simulink model "FlightControlArchitecture"  (R2022a)
settings: Solver=VariableStepAuto  StartTime=0.0  StopTime=10.0  RelTol=1e-3
settings Model: Creator=pownc  LastModifiedBy=pownc

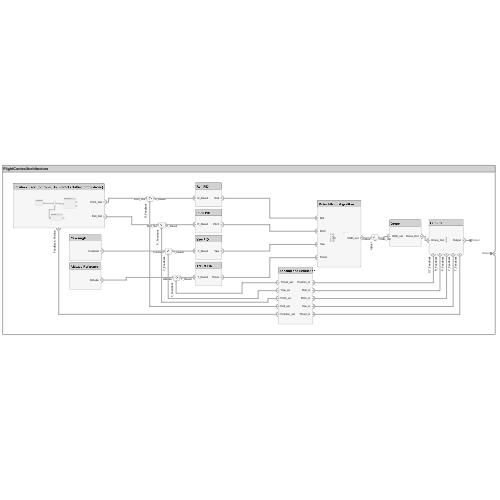
[thumbnail: Simulink's stored preview of the top-level diagram]
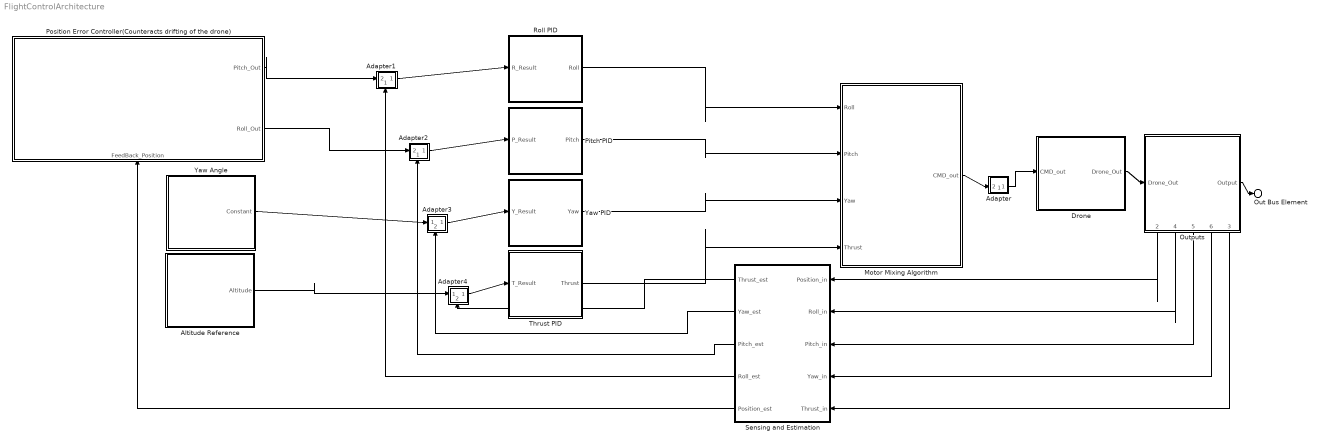
== system FlightControlArchitecture ==
  Adapter : Subsystem
      settings: PortSchema="{\"entries\":[{\"content\":{\"margin\":10,\"minimumSpacing\":15,\"sides\":[{\"content\":{\"connectorIds\":[\"In2\"]},\"type\":\"ConnectorPlacement.EquallySpacedRectSide\",\"uuid\":\"d6b19c1a-8540-4fb3-b3a7-b181a93e2dcd\"},{\"content\":{\"connectorIds\":[\"Out1\"],\"side\":\"RIGHT\"},\"type\":\"ConnectorPlacement.EquallySpacedRectSide\",\"uuid\":\"919fe610-1017-4d7e-ba89-b997ed30f941\"},{\"content\":{\"connectorIds\":[],\"side\":\"TOP\"},\"type\":\"ConnectorPlacement.EquallySpacedRectSide\",\"uuid\":\"6473f4db-e183-4279-8b70-07d1c7c027c3\"},{\"content\":{\"connectorIds\":[\"In1\"],\"side\":\"BOTTOM\"},\"type\":\"ConnectorPlacement.EquallySpacedRectSide\",\"uuid\":\"001743d6-53a9-4507-8ba9-ff0a8338509d\"}]},\"type\":\"ConnectorPlacement.EquallySpacedConnector\",\"uuid\":\"f0cd8fda-dd3e-48df-a1f9-a7820f464db5\"}],\"packageUris\":[\"http://schema.mathworks.com/mf0/Connector/R2020b\"],\"version\":\"1.0\"}"
  Adapter1 : Subsystem
      settings: PortSchema="{\"entries\":[{\"content\":{\"margin\":10,\"minimumSpacing\":15,\"sides\":[{\"content\":{\"connectorIds\":[\"In2\"]},\"type\":\"ConnectorPlacement.EquallySpacedRectSide\",\"uuid\":\"d6b19c1a-8540-4fb3-b3a7-b181a93e2dcd\"},{\"content\":{\"connectorIds\":[\"Out1\"],\"side\":\"RIGHT\"},\"type\":\"ConnectorPlacement.EquallySpacedRectSide\",\"uuid\":\"919fe610-1017-4d7e-ba89-b997ed30f941\"},{\"content\":{\"connectorIds\":[],\"side\":\"TOP\"},\"type\":\"ConnectorPlacement.EquallySpacedRectSide\",\"uuid\":\"6473f4db-e183-4279-8b70-07d1c7c027c3\"},{\"content\":{\"connectorIds\":[\"In1\"],\"side\":\"BOTTOM\"},\"type\":\"ConnectorPlacement.EquallySpacedRectSide\",\"uuid\":\"7437e3f3-5fc3-44ba-b792-8c2483ff9ea8\"}]},\"type\":\"ConnectorPlacement.EquallySpacedConnector\",\"uuid\":\"f0cd8fda-dd3e-48df-a1f9-a7820f464db5\"}],\"packageUris\":[\"http://schema.mathworks.com/mf0/Connector/R2020b\"],\"version\":\"1.0\"}"
  Adapter2 : Subsystem
      settings: PortSchema="{\"entries\":[{\"content\":{\"margin\":10,\"minimumSpacing\":15,\"sides\":[{\"content\":{\"connectorIds\":[\"In2\"]},\"type\":\"ConnectorPlacement.EquallySpacedRectSide\",\"uuid\":\"d6b19c1a-8540-4fb3-b3a7-b181a93e2dcd\"},{\"content\":{\"connectorIds\":[\"Out1\"],\"side\":\"RIGHT\"},\"type\":\"ConnectorPlacement.EquallySpacedRectSide\",\"uuid\":\"919fe610-1017-4d7e-ba89-b997ed30f941\"},{\"content\":{\"connectorIds\":[],\"side\":\"TOP\"},\"type\":\"ConnectorPlacement.EquallySpacedRectSide\",\"uuid\":\"6473f4db-e183-4279-8b70-07d1c7c027c3\"},{\"content\":{\"connectorIds\":[\"In1\"],\"side\":\"BOTTOM\"},\"type\":\"ConnectorPlacement.EquallySpacedRectSide\",\"uuid\":\"a3707513-231b-4166-bb59-f1312184589a\"}]},\"type\":\"ConnectorPlacement.EquallySpacedConnector\",\"uuid\":\"f0cd8fda-dd3e-48df-a1f9-a7820f464db5\"}],\"packageUris\":[\"http://schema.mathworks.com/mf0/Connector/R2020b\"],\"version\":\"1.0\"}"
  Adapter3 : Subsystem
      settings: PortSchema="{\"entries\":[{\"content\":{\"margin\":10,\"minimumSpacing\":15,\"sides\":[{\"content\":{\"connectorIds\":[\"In1\"]},\"type\":\"ConnectorPlacement.EquallySpacedRectSide\",\"uuid\":\"d6b19c1a-8540-4fb3-b3a7-b181a93e2dcd\"},{\"content\":{\"connectorIds\":[\"Out1\"],\"side\":\"RIGHT\"},\"type\":\"ConnectorPlacement.EquallySpacedRectSide\",\"uuid\":\"919fe610-1017-4d7e-ba89-b997ed30f941\"},{\"content\":{\"connectorIds\":[],\"side\":\"TOP\"},\"type\":\"ConnectorPlacement.EquallySpacedRectSide\",\"uuid\":\"6473f4db-e183-4279-8b70-07d1c7c027c3\"},{\"content\":{\"connectorIds\":[\"In2\"],\"side\":\"BOTTOM\"},\"type\":\"ConnectorPlacement.EquallySpacedRectSide\",\"uuid\":\"50c041b2-6c26-49b7-bedc-5dbf061703b8\"}]},\"type\":\"ConnectorPlacement.EquallySpacedConnector\",\"uuid\":\"f0cd8fda-dd3e-48df-a1f9-a7820f464db5\"}],\"packageUris\":[\"http://schema.mathworks.com/mf0/Connector/R2020b\"],\"version\":\"1.0\"}"
  Adapter4 : Subsystem
      settings: PortSchema="{\"entries\":[{\"content\":{\"margin\":10,\"minimumSpacing\":15,\"sides\":[{\"content\":{\"connectorIds\":[\"In1\"]},\"type\":\"ConnectorPlacement.EquallySpacedRectSide\",\"uuid\":\"d6b19c1a-8540-4fb3-b3a7-b181a93e2dcd\"},{\"content\":{\"connectorIds\":[\"Out1\"],\"side\":\"RIGHT\"},\"type\":\"ConnectorPlacement.EquallySpacedRectSide\",\"uuid\":\"919fe610-1017-4d7e-ba89-b997ed30f941\"},{\"content\":{\"connectorIds\":[],\"side\":\"TOP\"},\"type\":\"ConnectorPlacement.EquallySpacedRectSide\",\"uuid\":\"6473f4db-e183-4279-8b70-07d1c7c027c3\"},{\"content\":{\"connectorIds\":[\"In2\"],\"side\":\"BOTTOM\"},\"type\":\"ConnectorPlacement.EquallySpacedRectSide\",\"uuid\":\"d02c2b55-2766-4554-926c-619c29dbf015\"}]},\"type\":\"ConnectorPlacement.EquallySpacedConnector\",\"uuid\":\"f0cd8fda-dd3e-48df-a1f9-a7820f464db5\"}],\"packageUris\":[\"http://schema.mathworks.com/mf0/Connector/R2020b\"],\"version\":\"1.0\"}"
  Altitude Reference : Subsystem
      settings: PortSchema="{\"entries\":[{\"content\":{\"headerSize\":26,\"margin\":15,\"minimumSpacing\":25,\"sides\":[{\"content\":{\"connectorIds\":[]},\"type\":\"ConnectorPlacement.EquallySpacedRectSide\",\"uuid\":\"d6b19c1a-8540-4fb3-b3a7-b181a93e2dcd\"},{\"content\":{\"connectorIds\":[\"Out1\"],\"side\":\"RIGHT\"},\"type\":\"ConnectorPlacement.EquallySpacedRectSide\",\"uuid\":\"919fe610-1017-4d7e-ba89-b997ed30f941\"},{\"content\":{\"connectorIds\":[],\"side\":\"TOP\"},\"type\":\"ConnectorPlacement.EquallySpacedRectSide\",\"uuid\":\"6473f4db-e183-4279-8b70-07d1c7c027c3\"}]},\"type\":\"ConnectorPlacement.EquallySpacedConnector\",\"uuid\":\"f0cd8fda-dd3e-48df-a1f9-a7820f464db5\"}],\"packageUris\":[\"http://schema.mathworks.com/mf0/Connector/R2020b\"],\"version\":\"1.0\"}"
  Drone : Subsystem
      settings: PortSchema="{\"entries\":[{\"content\":{\"headerSize\":26,\"margin\":15,\"minimumSpacing\":25,\"sides\":[{\"content\":{\"connectorIds\":[\"In1\"]},\"type\":\"ConnectorPlacement.EquallySpacedRectSide\",\"uuid\":\"d6b19c1a-8540-4fb3-b3a7-b181a93e2dcd\"},{\"content\":{\"connectorIds\":[\"Out1\"],\"side\":\"RIGHT\"},\"type\":\"ConnectorPlacement.EquallySpacedRectSide\",\"uuid\":\"919fe610-1017-4d7e-ba89-b997ed30f941\"},{\"content\":{\"connectorIds\":[],\"side\":\"TOP\"},\"type\":\"ConnectorPlacement.EquallySpacedRectSide\",\"uuid\":\"6473f4db-e183-4279-8b70-07d1c7c027c3\"}]},\"type\":\"ConnectorPlacement.EquallySpacedConnector\",\"uuid\":\"f0cd8fda-dd3e-48df-a1f9-a7820f464db5\"}],\"packageUris\":[\"http://schema.mathworks.com/mf0/Connector/R2020b\"],\"version\":\"1.0\"}"
  Motor Mixing Algorithm : Subsystem
      settings: PortSchema="{\"entries\":[{\"content\":{\"headerSize\":26,\"margin\":15,\"minimumSpacing\":25,\"sides\":[{\"content\":{\"connectorIds\":[\"In1\",\"In2\",\"In3\",\"In4\"]},\"type\":\"ConnectorPlacement.EquallySpacedRectSide\",\"uuid\":\"7a3b38b8-6f09-4e2e-ab1c-f7a95debc383\"},{\"content\":{\"connectorIds\":[\"Out1\"],\"side\":\"RIGHT\"},\"type\":\"ConnectorPlacement.EquallySpacedRectSide\",\"uuid\":\"c60604c7-2225-45b1-bf81-c4b0e619cd15\"},{\"content\":{\"connectorIds\":[],\"side\":\"TOP\"},\"type\":\"ConnectorPlacement.EquallySpacedRectSide\",\"uuid\":\"851cd2f2-1711-4180-941f-21dd02fa4550\"}]},\"type\":\"ConnectorPlacement.EquallySpacedConnector\",\"uuid\":\"5057f251-a455-43c7-b15c-b3d1f8a9e1a3\"}],\"packageUris\":[\"http://schema.mathworks.com/mf0/Connector/R2020b\"],\"version\":\"1.0\"}"
  Outputs : Subsystem
      settings: PortSchema="{\"entries\":[{\"content\":{\"headerSize\":26,\"margin\":15,\"minimumSpacing\":25,\"sides\":[{\"content\":{\"connectorIds\":[\"In1\"]},\"type\":\"ConnectorPlacement.EquallySpacedRectSide\",\"uuid\":\"d6b19c1a-8540-4fb3-b3a7-b181a93e2dcd\"},{\"content\":{\"connectorIds\":[\"Out1\"],\"side\":\"RIGHT\"},\"type\":\"ConnectorPlacement.EquallySpacedRectSide\",\"uuid\":\"919fe610-1017-4d7e-ba89-b997ed30f941\"},{\"content\":{\"connectorIds\":[],\"side\":\"TOP\"},\"type\":\"ConnectorPlacement.EquallySpacedRectSide\",\"uuid\":\"6473f4db-e183-4279-8b70-07d1c7c027c3\"},{\"content\":{\"connectorIds\":[\"Out2\",\"Out4\",\"Out5\",\"Out6\",\"Out3\"],\"side\":\"BOTTOM\"},\"type\":\"ConnectorPlacement.EquallySpacedRectSide\",\"uuid\":\"c79be452-f41b-4e6d-ad81-53eba8a6a323\"}]},\"type\":\"ConnectorPlacement.EquallySpacedConnector\",\"uuid\":\"f0cd8fda-dd3e-48df-a1f9-a7820f464db5\"}],\"packageUris\":[\"http://schema.mathworks.com/mf0/Connector/R2020b\"],\"version\":\"1.0\"}"
  Pitch PID : Subsystem
      settings: PortSchema="{\"entries\":[{\"content\":{\"headerSize\":26,\"margin\":15,\"minimumSpacing\":25,\"sides\":[{\"content\":{\"connectorIds\":[\"In1\"]},\"type\":\"ConnectorPlacement.EquallySpacedRectSide\",\"uuid\":\"d6b19c1a-8540-4fb3-b3a7-b181a93e2dcd\"},{\"content\":{\"connectorIds\":[\"Out1\"],\"side\":\"RIGHT\"},\"type\":\"ConnectorPlacement.EquallySpacedRectSide\",\"uuid\":\"919fe610-1017-4d7e-ba89-b997ed30f941\"},{\"content\":{\"connectorIds\":[],\"side\":\"TOP\"},\"type\":\"ConnectorPlacement.EquallySpacedRectSide\",\"uuid\":\"6473f4db-e183-4279-8b70-07d1c7c027c3\"}]},\"type\":\"ConnectorPlacement.EquallySpacedConnector\",\"uuid\":\"f0cd8fda-dd3e-48df-a1f9-a7820f464db5\"}],\"packageUris\":[\"http://schema.mathworks.com/mf0/Connector/R2020b\"],\"version\":\"1.0\"}"
  Position Error Controller(Counteracts drifting of the drone) : Subsystem
      settings: PortSchema="{\"entries\":[{\"content\":{\"headerSize\":26,\"margin\":15,\"minimumSpacing\":25,\"sides\":[{\"content\":{\"connectorIds\":[]},\"type\":\"ConnectorPlacement.EquallySpacedRectSide\",\"uuid\":\"d6b19c1a-8540-4fb3-b3a7-b181a93e2dcd\"},{\"content\":{\"connectorIds\":[\"Out1\",\"Out2\"],\"side\":\"RIGHT\"},\"type\":\"ConnectorPlacement.EquallySpacedRectSide\",\"uuid\":\"919fe610-1017-4d7e-ba89-b997ed30f941\"},{\"content\":{\"connectorIds\":[],\"side\":\"TOP\"},\"type\":\"ConnectorPlacement.EquallySpacedRectSide\",\"uuid\":\"6473f4db-e183-4279-8b70-07d1c7c027c3\"},{\"content\":{\"connectorIds\":[\"In1\"],\"side\":\"BOTTOM\"},\"type\":\"ConnectorPlacement.EquallySpacedRectSide\",\"uuid\":\"7201be1c-4784-47e8-b556-a6345fcdd719\"}]},\"type\":\"ConnectorPlacement.EquallySpacedConnector\",\"uuid\":\"f0cd8fda-dd3e-48df-a1f9-a7820f464db5\"}],\"packageUris\":[\"http://schema.mathworks.com/mf0/Connector/R2020b\"],\"version\":\"1.0\"}"
  Roll PID : Subsystem
      settings: PortSchema="{\"entries\":[{\"content\":{\"headerSize\":26,\"margin\":15,\"minimumSpacing\":25,\"sides\":[{\"content\":{\"connectorIds\":[\"In1\"]},\"type\":\"ConnectorPlacement.EquallySpacedRectSide\",\"uuid\":\"d6b19c1a-8540-4fb3-b3a7-b181a93e2dcd\"},{\"content\":{\"connectorIds\":[\"Out1\"],\"side\":\"RIGHT\"},\"type\":\"ConnectorPlacement.EquallySpacedRectSide\",\"uuid\":\"919fe610-1017-4d7e-ba89-b997ed30f941\"},{\"content\":{\"connectorIds\":[],\"side\":\"TOP\"},\"type\":\"ConnectorPlacement.EquallySpacedRectSide\",\"uuid\":\"6473f4db-e183-4279-8b70-07d1c7c027c3\"}]},\"type\":\"ConnectorPlacement.EquallySpacedConnector\",\"uuid\":\"f0cd8fda-dd3e-48df-a1f9-a7820f464db5\"}],\"packageUris\":[\"http://schema.mathworks.com/mf0/Connector/R2020b\"],\"version\":\"1.0\"}"
  Sensing and Estimation : Subsystem
      settings: PortSchema="{\"entries\":[{\"content\":{\"headerSize\":26,\"margin\":15,\"minimumSpacing\":25,\"sides\":[{\"content\":{\"connectorIds\":[\"Out1\",\"Out2\",\"Out3\",\"Out4\",\"Out5\"]},\"type\":\"ConnectorPlacement.EquallySpacedRectSide\",\"uuid\":\"d6b19c1a-8540-4fb3-b3a7-b181a93e2dcd\"},{\"content\":{\"connectorIds\":[\"In5\",\"In4\",\"In3\",\"In2\",\"In1\"],\"side\":\"RIGHT\"},\"type\":\"ConnectorPlacement.EquallySpacedRectSide\",\"uuid\":\"919fe610-1017-4d7e-ba89-b997ed30f941\"},{\"content\":{\"connectorIds\":[],\"side\":\"TOP\"},\"type\":\"ConnectorPlacement.EquallySpacedRectSide\",\"uuid\":\"6473f4db-e183-4279-8b70-07d1c7c027c3\"}]},\"type\":\"ConnectorPlacement.EquallySpacedConnector\",\"uuid\":\"f0cd8fda-dd3e-48df-a1f9-a7820f464db5\"}],\"packageUris\":[\"http://schema.mathworks.com/mf0/Connector/R2020b\"],\"version\":\"1.0\"}"
  Thrust PID : Subsystem
      settings: PortSchema="{\"entries\":[{\"content\":{\"headerSize\":26,\"margin\":15,\"minimumSpacing\":25,\"sides\":[{\"content\":{\"connectorIds\":[\"In1\"]},\"type\":\"ConnectorPlacement.EquallySpacedRectSide\",\"uuid\":\"d6b19c1a-8540-4fb3-b3a7-b181a93e2dcd\"},{\"content\":{\"connectorIds\":[\"Out1\"],\"side\":\"RIGHT\"},\"type\":\"ConnectorPlacement.EquallySpacedRectSide\",\"uuid\":\"919fe610-1017-4d7e-ba89-b997ed30f941\"},{\"content\":{\"connectorIds\":[],\"side\":\"TOP\"},\"type\":\"ConnectorPlacement.EquallySpacedRectSide\",\"uuid\":\"6473f4db-e183-4279-8b70-07d1c7c027c3\"}]},\"type\":\"ConnectorPlacement.EquallySpacedConnector\",\"uuid\":\"f0cd8fda-dd3e-48df-a1f9-a7820f464db5\"}],\"packageUris\":[\"http://schema.mathworks.com/mf0/Connector/R2020b\"],\"version\":\"1.0\"}"
  Yaw Angle : Subsystem
      settings: PortSchema="{\"entries\":[{\"content\":{\"headerSize\":26,\"margin\":15,\"minimumSpacing\":25,\"sides\":[{\"content\":{\"connectorIds\":[]},\"type\":\"ConnectorPlacement.EquallySpacedRectSide\",\"uuid\":\"d6b19c1a-8540-4fb3-b3a7-b181a93e2dcd\"},{\"content\":{\"connectorIds\":[\"Out1\"],\"side\":\"RIGHT\"},\"type\":\"ConnectorPlacement.EquallySpacedRectSide\",\"uuid\":\"919fe610-1017-4d7e-ba89-b997ed30f941\"},{\"content\":{\"connectorIds\":[],\"side\":\"TOP\"},\"type\":\"ConnectorPlacement.EquallySpacedRectSide\",\"uuid\":\"6473f4db-e183-4279-8b70-07d1c7c027c3\"}]},\"type\":\"ConnectorPlacement.EquallySpacedConnector\",\"uuid\":\"f0cd8fda-dd3e-48df-a1f9-a7820f464db5\"}],\"packageUris\":[\"http://schema.mathworks.com/mf0/Connector/R2020b\"],\"version\":\"1.0\"}"
  Yaw PID : Subsystem
      settings: PortSchema="{\"entries\":[{\"content\":{\"headerSize\":26,\"margin\":15,\"minimumSpacing\":25,\"sides\":[{\"content\":{\"connectorIds\":[\"In1\"]},\"type\":\"ConnectorPlacement.EquallySpacedRectSide\",\"uuid\":\"d6b19c1a-8540-4fb3-b3a7-b181a93e2dcd\"},{\"content\":{\"connectorIds\":[\"Out1\"],\"side\":\"RIGHT\"},\"type\":\"ConnectorPlacement.EquallySpacedRectSide\",\"uuid\":\"919fe610-1017-4d7e-ba89-b997ed30f941\"},{\"content\":{\"connectorIds\":[],\"side\":\"TOP\"},\"type\":\"ConnectorPlacement.EquallySpacedRectSide\",\"uuid\":\"6473f4db-e183-4279-8b70-07d1c7c027c3\"}]},\"type\":\"ConnectorPlacement.EquallySpacedConnector\",\"uuid\":\"f0cd8fda-dd3e-48df-a1f9-a7820f464db5\"}],\"packageUris\":[\"http://schema.mathworks.com/mf0/Connector/R2020b\"],\"version\":\"1.0\"}"
  Out Bus Element : Outport  PortName=Output
  wires:
  Roll PID/1(Roll) -> Motor Mixing Algorithm/1(Roll)
  Pitch PID/1(Pitch) -> Motor Mixing Algorithm/2(Pitch)
  Yaw PID/1(Yaw) -> Motor Mixing Algorithm/3(Yaw)
  Thrust PID/1(Thrust) -> Motor Mixing Algorithm/4(Thrust)
  Adapter/1(CMD_out) -> Drone/1(CMD_out)
  Motor Mixing Algorithm/1(CMD_out) -> Adapter/2(InBus)
  Position Error Controller(Counteracts drifting of the drone)/1(Pitch_Out) -> Adapter1/2(Pitch_Out)
  Drone/1(Drone_Out) -> Outputs/1(Drone_Out)
  Adapter4/1(T_Result) -> Thrust PID/1(T_Result)
  Position Error Controller(Counteracts drifting of the drone)/2(Roll_Out) -> Adapter2/2(Roll_Out)
  Adapter1/1(R_Result) -> Roll PID/1(R_Result)
  Adapter2/1(P_Result) -> Pitch PID/1(P_Result)
  Adapter3/1(Y_Result) -> Yaw PID/1(Y_Result)
  Outputs/1(Output) -> Out Bus Element/1
  Outputs/2(XY_Feedback) -> Sensing and Estimation/5(Position_in)
  Outputs/4(R_Feedback) -> Sensing and Estimation/4(Roll_in)
  Outputs/5(P_Feedback) -> Sensing and Estimation/3(Pitch_in)
  Outputs/6(Y_Feedback) -> Sensing and Estimation/2(Yaw_in)
  Outputs/3(T_Feedback) -> Sensing and Estimation/1(Thrust_in)
  Sensing and Estimation/1(Thrust_est) -> Adapter4/2(T_Feedback)
  Sensing and Estimation/2(Yaw_est) -> Adapter3/2(Y_Feedback)
  Sensing and Estimation/3(Pitch_est) -> Adapter2/1(P_Feedback)
  Sensing and Estimation/4(Roll_est) -> Adapter1/1(R_Feedback)
  Sensing and Estimation/5(Position_est) -> Position Error Controller(Counteracts drifting of the drone)/1(FeedBack_Position)
  Yaw Angle/1(Constant) -> Adapter3/1(Constant)
  Altitude Reference/1(Altitude) -> Adapter4/1(Altitude)

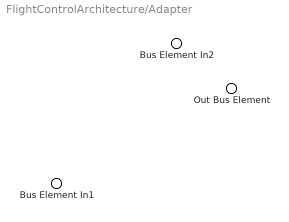
== system FlightControlArchitecture/Adapter ==
  Bus Element In2 : Inport  PortName=InBus1
  Bus Element In1 : Inport  Port=2  PortName=InBus
  Out Bus Element : Outport  PortName=CMD_out

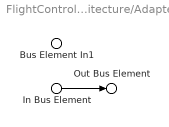
== system FlightControlArchitecture/Adapter1 ==
  Bus Element In1 : Inport  PortName=R_Feedback
  In Bus Element : Inport  Port=2  PortName=Pitch_Out
  Out Bus Element : Outport  PortName=R_Result
  wires:
  In Bus Element/1 -> Out Bus Element/1

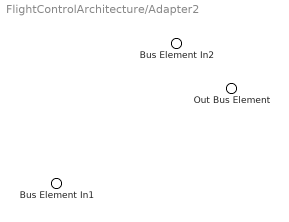
== system FlightControlArchitecture/Adapter2 ==
  Bus Element In2 : Inport  PortName=P_Feedback
  Bus Element In1 : Inport  Port=2  PortName=Roll_Out
  Out Bus Element : Outport  PortName=P_Result

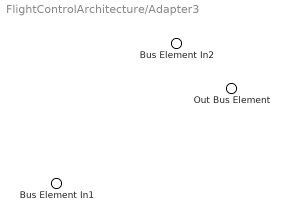
== system FlightControlArchitecture/Adapter3 ==
  Bus Element In2 : Inport  PortName=Constant
  Bus Element In1 : Inport  Port=2  PortName=Y_Feedback
  Out Bus Element : Outport  PortName=Y_Result

== system FlightControlArchitecture/Adapter4 ==
  Bus Element In2 : Inport  PortName=Altitude
  Bus Element In1 : Inport  Port=2  PortName=T_Feedback
  Out Bus Element : Outport  PortName=T_Result

== system FlightControlArchitecture/Altitude Reference ==
  Bus Element Out1 : Outport  PortName=Altitude

== system FlightControlArchitecture/Drone ==
  Bus Element In1 : Inport  PortName=CMD_out
  Bus Element Out1 : Outport  PortName=Drone_Out

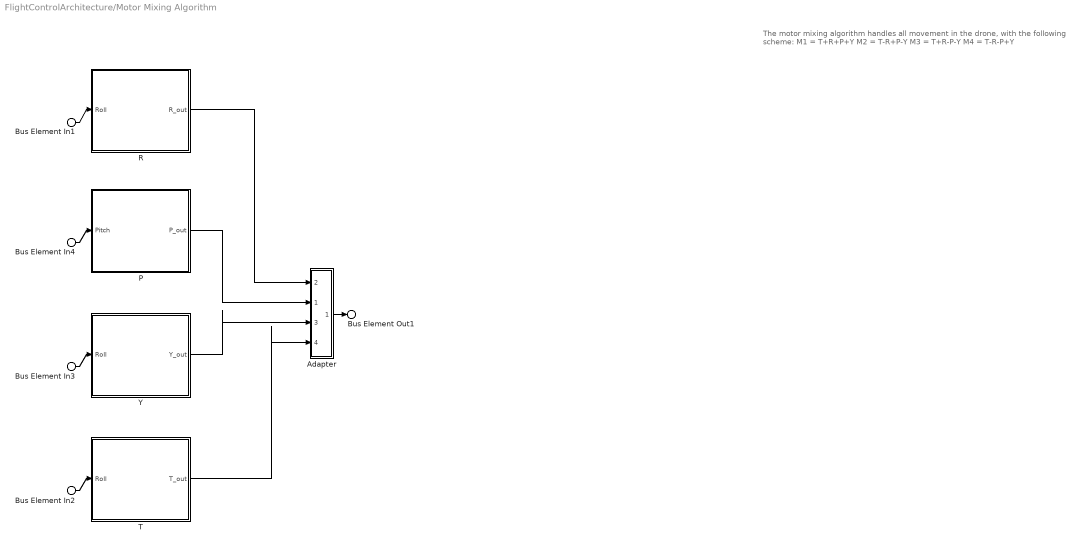
== system FlightControlArchitecture/Motor Mixing Algorithm ==
  note: The motor mixing algorithm handles all
      | movement in the drone, with the following
      | scheme:
      |
      | M1 = T+R+P+Y
      | M2 = T-R+P-Y
      | M3 = T+R-P-Y
      | M4 = T-R-P+Y
  Bus Element In1 : Inport  PortName=Roll
  Bus Element In4 : Inport  Port=2  PortName=Pitch
  Bus Element In3 : Inport  Port=3  PortName=Yaw
  Bus Element In2 : Inport  Port=4  PortName=Thrust
  Adapter : Subsystem
      settings: PortSchema="{\"entries\":[{\"content\":{\"margin\":10,\"minimumSpacing\":15,\"sides\":[{\"content\":{\"connectorIds\":[\"In2\",\"In1\",\"In3\",\"In4\"]},\"type\":\"ConnectorPlacement.EquallySpacedRectSide\",\"uuid\":\"7a3b38b8-6f09-4e2e-ab1c-f7a95debc383\"},{\"content\":{\"connectorIds\":[\"Out1\"],\"side\":\"RIGHT\"},\"type\":\"ConnectorPlacement.EquallySpacedRectSide\",\"uuid\":\"c60604c7-2225-45b1-bf81-c4b0e619cd15\"},{\"content\":{\"connectorIds\":[],\"side\":\"TOP\"},\"type\":\"ConnectorPlacement.EquallySpacedRectSide\",\"uuid\":\"851cd2f2-1711-4180-941f-21dd02fa4550\"},{\"content\":{\"connectorIds\":[],\"side\":\"BOTTOM\"},\"type\":\"ConnectorPlacement.EquallySpacedRectSide\",\"uuid\":\"a4badc9f-aa9e-49e4-ad30-e5b76d116eb5\"}]},\"type\":\"ConnectorPlacement.EquallySpacedConnector\",\"uuid\":\"5057f251-a455-43c7-b15c-b3d1f8a9e1a3\"}],\"packageUris\":[\"http://schema.mathworks.com/mf0/Connector/R2020b\"],\"version\":\"1.0\"}"
  P : Subsystem
      settings: PortSchema="{\"entries\":[{\"content\":{\"headerSize\":26,\"margin\":15,\"minimumSpacing\":25,\"sides\":[{\"content\":{\"connectorIds\":[\"In1\"]},\"type\":\"ConnectorPlacement.EquallySpacedRectSide\",\"uuid\":\"7a3b38b8-6f09-4e2e-ab1c-f7a95debc383\"},{\"content\":{\"connectorIds\":[\"Out1\"],\"side\":\"RIGHT\"},\"type\":\"ConnectorPlacement.EquallySpacedRectSide\",\"uuid\":\"c60604c7-2225-45b1-bf81-c4b0e619cd15\"},{\"content\":{\"connectorIds\":[],\"side\":\"TOP\"},\"type\":\"ConnectorPlacement.EquallySpacedRectSide\",\"uuid\":\"851cd2f2-1711-4180-941f-21dd02fa4550\"}]},\"type\":\"ConnectorPlacement.EquallySpacedConnector\",\"uuid\":\"5057f251-a455-43c7-b15c-b3d1f8a9e1a3\"}],\"packageUris\":[\"http://schema.mathworks.com/mf0/Connector/R2020b\"],\"version\":\"1.0\"}"
  R : Subsystem
      settings: PortSchema="{\"entries\":[{\"content\":{\"headerSize\":26,\"margin\":15,\"minimumSpacing\":25,\"sides\":[{\"content\":{\"connectorIds\":[\"In1\"]},\"type\":\"ConnectorPlacement.EquallySpacedRectSide\",\"uuid\":\"7a3b38b8-6f09-4e2e-ab1c-f7a95debc383\"},{\"content\":{\"connectorIds\":[\"Out1\"],\"side\":\"RIGHT\"},\"type\":\"ConnectorPlacement.EquallySpacedRectSide\",\"uuid\":\"c60604c7-2225-45b1-bf81-c4b0e619cd15\"},{\"content\":{\"connectorIds\":[],\"side\":\"TOP\"},\"type\":\"ConnectorPlacement.EquallySpacedRectSide\",\"uuid\":\"851cd2f2-1711-4180-941f-21dd02fa4550\"}]},\"type\":\"ConnectorPlacement.EquallySpacedConnector\",\"uuid\":\"5057f251-a455-43c7-b15c-b3d1f8a9e1a3\"}],\"packageUris\":[\"http://schema.mathworks.com/mf0/Connector/R2020b\"],\"version\":\"1.0\"}"
  T : Subsystem
      settings: PortSchema="{\"entries\":[{\"content\":{\"headerSize\":26,\"margin\":15,\"minimumSpacing\":25,\"sides\":[{\"content\":{\"connectorIds\":[\"In1\"]},\"type\":\"ConnectorPlacement.EquallySpacedRectSide\",\"uuid\":\"7a3b38b8-6f09-4e2e-ab1c-f7a95debc383\"},{\"content\":{\"connectorIds\":[\"Out1\"],\"side\":\"RIGHT\"},\"type\":\"ConnectorPlacement.EquallySpacedRectSide\",\"uuid\":\"c60604c7-2225-45b1-bf81-c4b0e619cd15\"},{\"content\":{\"connectorIds\":[],\"side\":\"TOP\"},\"type\":\"ConnectorPlacement.EquallySpacedRectSide\",\"uuid\":\"851cd2f2-1711-4180-941f-21dd02fa4550\"}]},\"type\":\"ConnectorPlacement.EquallySpacedConnector\",\"uuid\":\"5057f251-a455-43c7-b15c-b3d1f8a9e1a3\"}],\"packageUris\":[\"http://schema.mathworks.com/mf0/Connector/R2020b\"],\"version\":\"1.0\"}"
  Y : Subsystem
      settings: PortSchema="{\"entries\":[{\"content\":{\"headerSize\":26,\"margin\":15,\"minimumSpacing\":25,\"sides\":[{\"content\":{\"connectorIds\":[\"In1\"]},\"type\":\"ConnectorPlacement.EquallySpacedRectSide\",\"uuid\":\"7a3b38b8-6f09-4e2e-ab1c-f7a95debc383\"},{\"content\":{\"connectorIds\":[\"Out1\"],\"side\":\"RIGHT\"},\"type\":\"ConnectorPlacement.EquallySpacedRectSide\",\"uuid\":\"c60604c7-2225-45b1-bf81-c4b0e619cd15\"},{\"content\":{\"connectorIds\":[],\"side\":\"TOP\"},\"type\":\"ConnectorPlacement.EquallySpacedRectSide\",\"uuid\":\"851cd2f2-1711-4180-941f-21dd02fa4550\"}]},\"type\":\"ConnectorPlacement.EquallySpacedConnector\",\"uuid\":\"5057f251-a455-43c7-b15c-b3d1f8a9e1a3\"}],\"packageUris\":[\"http://schema.mathworks.com/mf0/Connector/R2020b\"],\"version\":\"1.0\"}"
  Bus Element Out1 : Outport  PortName=CMD_out
  wires:
  Bus Element In1/1 -> R/1(Roll)
  Bus Element In2/1 -> T/1(Roll)
  Bus Element In3/1 -> Y/1(Roll)
  Bus Element In4/1 -> P/1(Pitch)
  P/1(P_out) -> Adapter/1(P_out)
  R/1(R_out) -> Adapter/2(R_out)
  Y/1(Y_out) -> Adapter/3(Y_out)
  T/1(T_out) -> Adapter/4(T_out)
  Adapter/1(CMD_out) -> Bus Element Out1/1

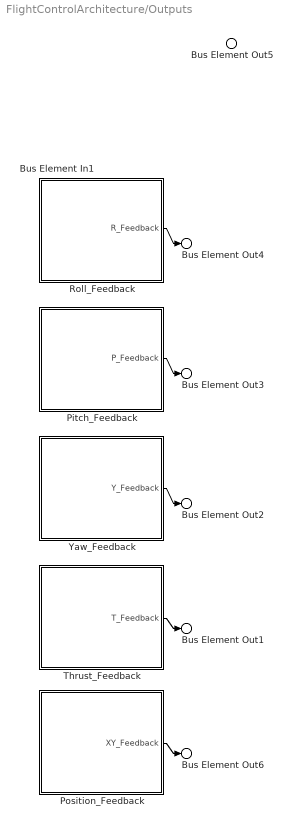
== system FlightControlArchitecture/Outputs ==
  Bus Element In1 : Inport  PortName=Drone_Out
  Pitch_Feedback : Subsystem
      settings: PortSchema="{\"entries\":[{\"content\":{\"headerSize\":26,\"margin\":15,\"minimumSpacing\":25,\"sides\":[{\"content\":{\"connectorIds\":[]},\"type\":\"ConnectorPlacement.EquallySpacedRectSide\",\"uuid\":\"d6b19c1a-8540-4fb3-b3a7-b181a93e2dcd\"},{\"content\":{\"connectorIds\":[\"Out1\"],\"side\":\"RIGHT\"},\"type\":\"ConnectorPlacement.EquallySpacedRectSide\",\"uuid\":\"919fe610-1017-4d7e-ba89-b997ed30f941\"},{\"content\":{\"connectorIds\":[],\"side\":\"TOP\"},\"type\":\"ConnectorPlacement.EquallySpacedRectSide\",\"uuid\":\"6473f4db-e183-4279-8b70-07d1c7c027c3\"}]},\"type\":\"ConnectorPlacement.EquallySpacedConnector\",\"uuid\":\"f0cd8fda-dd3e-48df-a1f9-a7820f464db5\"}],\"packageUris\":[\"http://schema.mathworks.com/mf0/Connector/R2020b\"],\"version\":\"1.0\"}"
  Position_Feedback : Subsystem
      settings: PortSchema="{\"entries\":[{\"content\":{\"headerSize\":26,\"margin\":15,\"minimumSpacing\":25,\"sides\":[{\"content\":{\"connectorIds\":[]},\"type\":\"ConnectorPlacement.EquallySpacedRectSide\",\"uuid\":\"d6b19c1a-8540-4fb3-b3a7-b181a93e2dcd\"},{\"content\":{\"connectorIds\":[\"Out1\"],\"side\":\"RIGHT\"},\"type\":\"ConnectorPlacement.EquallySpacedRectSide\",\"uuid\":\"919fe610-1017-4d7e-ba89-b997ed30f941\"},{\"content\":{\"connectorIds\":[],\"side\":\"TOP\"},\"type\":\"ConnectorPlacement.EquallySpacedRectSide\",\"uuid\":\"6473f4db-e183-4279-8b70-07d1c7c027c3\"}]},\"type\":\"ConnectorPlacement.EquallySpacedConnector\",\"uuid\":\"f0cd8fda-dd3e-48df-a1f9-a7820f464db5\"}],\"packageUris\":[\"http://schema.mathworks.com/mf0/Connector/R2020b\"],\"version\":\"1.0\"}"
  Roll_Feedback : Subsystem
      settings: PortSchema="{\"entries\":[{\"content\":{\"headerSize\":26,\"margin\":15,\"minimumSpacing\":25,\"sides\":[{\"content\":{\"connectorIds\":[]},\"type\":\"ConnectorPlacement.EquallySpacedRectSide\",\"uuid\":\"d6b19c1a-8540-4fb3-b3a7-b181a93e2dcd\"},{\"content\":{\"connectorIds\":[\"Out1\"],\"side\":\"RIGHT\"},\"type\":\"ConnectorPlacement.EquallySpacedRectSide\",\"uuid\":\"919fe610-1017-4d7e-ba89-b997ed30f941\"},{\"content\":{\"connectorIds\":[],\"side\":\"TOP\"},\"type\":\"ConnectorPlacement.EquallySpacedRectSide\",\"uuid\":\"6473f4db-e183-4279-8b70-07d1c7c027c3\"}]},\"type\":\"ConnectorPlacement.EquallySpacedConnector\",\"uuid\":\"f0cd8fda-dd3e-48df-a1f9-a7820f464db5\"}],\"packageUris\":[\"http://schema.mathworks.com/mf0/Connector/R2020b\"],\"version\":\"1.0\"}"
  Thrust_Feedback : Subsystem
      settings: PortSchema="{\"entries\":[{\"content\":{\"headerSize\":26,\"margin\":15,\"minimumSpacing\":25,\"sides\":[{\"content\":{\"connectorIds\":[]},\"type\":\"ConnectorPlacement.EquallySpacedRectSide\",\"uuid\":\"d6b19c1a-8540-4fb3-b3a7-b181a93e2dcd\"},{\"content\":{\"connectorIds\":[\"Out1\"],\"side\":\"RIGHT\"},\"type\":\"ConnectorPlacement.EquallySpacedRectSide\",\"uuid\":\"919fe610-1017-4d7e-ba89-b997ed30f941\"},{\"content\":{\"connectorIds\":[],\"side\":\"TOP\"},\"type\":\"ConnectorPlacement.EquallySpacedRectSide\",\"uuid\":\"6473f4db-e183-4279-8b70-07d1c7c027c3\"}]},\"type\":\"ConnectorPlacement.EquallySpacedConnector\",\"uuid\":\"f0cd8fda-dd3e-48df-a1f9-a7820f464db5\"}],\"packageUris\":[\"http://schema.mathworks.com/mf0/Connector/R2020b\"],\"version\":\"1.0\"}"
  Yaw_Feedback : Subsystem
      settings: PortSchema="{\"entries\":[{\"content\":{\"headerSize\":26,\"margin\":15,\"minimumSpacing\":25,\"sides\":[{\"content\":{\"connectorIds\":[]},\"type\":\"ConnectorPlacement.EquallySpacedRectSide\",\"uuid\":\"d6b19c1a-8540-4fb3-b3a7-b181a93e2dcd\"},{\"content\":{\"connectorIds\":[\"Out1\"],\"side\":\"RIGHT\"},\"type\":\"ConnectorPlacement.EquallySpacedRectSide\",\"uuid\":\"919fe610-1017-4d7e-ba89-b997ed30f941\"},{\"content\":{\"connectorIds\":[],\"side\":\"TOP\"},\"type\":\"ConnectorPlacement.EquallySpacedRectSide\",\"uuid\":\"6473f4db-e183-4279-8b70-07d1c7c027c3\"}]},\"type\":\"ConnectorPlacement.EquallySpacedConnector\",\"uuid\":\"f0cd8fda-dd3e-48df-a1f9-a7820f464db5\"}],\"packageUris\":[\"http://schema.mathworks.com/mf0/Connector/R2020b\"],\"version\":\"1.0\"}"
  Bus Element Out5 : Outport  PortName=Output
  Bus Element Out6 : Outport  Port=2  PortName=XY_Feedback
  Bus Element Out1 : Outport  Port=3  PortName=T_Feedback
  Bus Element Out4 : Outport  Port=4  PortName=R_Feedback
  Bus Element Out3 : Outport  Port=5  PortName=P_Feedback
  Bus Element Out2 : Outport  Port=6  PortName=Y_Feedback
  wires:
  Thrust_Feedback/1(T_Feedback) -> Bus Element Out1/1
  Yaw_Feedback/1(Y_Feedback) -> Bus Element Out2/1
  Pitch_Feedback/1(P_Feedback) -> Bus Element Out3/1
  Roll_Feedback/1(R_Feedback) -> Bus Element Out4/1
  Position_Feedback/1(XY_Feedback) -> Bus Element Out6/1

== system FlightControlArchitecture/Pitch PID ==
  Bus Element In1 : Inport  PortName=P_Result
  Bus Element Out1 : Outport  PortName=Pitch

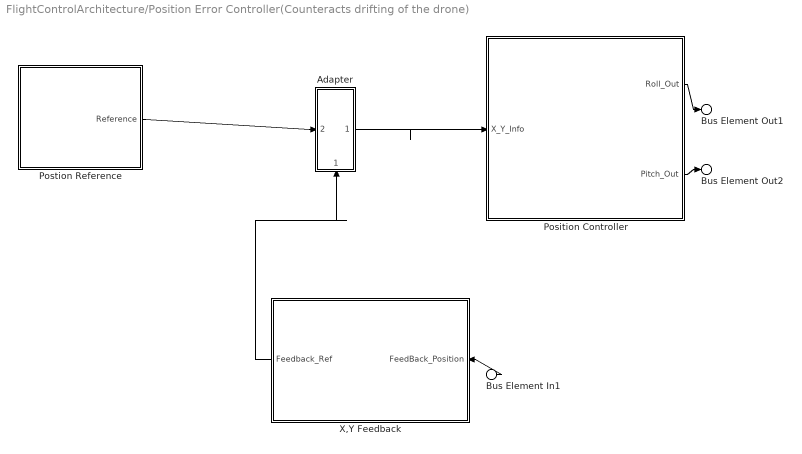
== system FlightControlArchitecture/Position Error Controller(Counteracts drifting of the drone) ==
  Bus Element In1 : Inport  PortName=FeedBack_Position
  Adapter : Subsystem
      settings: PortSchema="{\"entries\":[{\"content\":{\"margin\":10,\"minimumSpacing\":15,\"sides\":[{\"content\":{\"connectorIds\":[\"In2\"]},\"type\":\"ConnectorPlacement.EquallySpacedRectSide\",\"uuid\":\"d6b19c1a-8540-4fb3-b3a7-b181a93e2dcd\"},{\"content\":{\"connectorIds\":[\"Out1\"],\"side\":\"RIGHT\"},\"type\":\"ConnectorPlacement.EquallySpacedRectSide\",\"uuid\":\"919fe610-1017-4d7e-ba89-b997ed30f941\"},{\"content\":{\"connectorIds\":[],\"side\":\"TOP\"},\"type\":\"ConnectorPlacement.EquallySpacedRectSide\",\"uuid\":\"6473f4db-e183-4279-8b70-07d1c7c027c3\"},{\"content\":{\"connectorIds\":[\"In1\"],\"side\":\"BOTTOM\"},\"type\":\"ConnectorPlacement.EquallySpacedRectSide\",\"uuid\":\"a3cad288-231c-4860-82f0-66af71fff573\"}]},\"type\":\"ConnectorPlacement.EquallySpacedConnector\",\"uuid\":\"f0cd8fda-dd3e-48df-a1f9-a7820f464db5\"}],\"packageUris\":[\"http://schema.mathworks.com/mf0/Connector/R2020b\"],\"version\":\"1.0\"}"
  Position Controller : Subsystem
      settings: PortSchema="{\"entries\":[{\"content\":{\"headerSize\":26,\"margin\":15,\"minimumSpacing\":25,\"sides\":[{\"content\":{\"connectorIds\":[\"In1\"]},\"type\":\"ConnectorPlacement.EquallySpacedRectSide\",\"uuid\":\"d6b19c1a-8540-4fb3-b3a7-b181a93e2dcd\"},{\"content\":{\"connectorIds\":[\"Out1\",\"Out2\"],\"side\":\"RIGHT\"},\"type\":\"ConnectorPlacement.EquallySpacedRectSide\",\"uuid\":\"919fe610-1017-4d7e-ba89-b997ed30f941\"},{\"content\":{\"connectorIds\":[],\"side\":\"TOP\"},\"type\":\"ConnectorPlacement.EquallySpacedRectSide\",\"uuid\":\"6473f4db-e183-4279-8b70-07d1c7c027c3\"}]},\"type\":\"ConnectorPlacement.EquallySpacedConnector\",\"uuid\":\"f0cd8fda-dd3e-48df-a1f9-a7820f464db5\"}],\"packageUris\":[\"http://schema.mathworks.com/mf0/Connector/R2020b\"],\"version\":\"1.0\"}"
  Postion Reference : Subsystem
      settings: PortSchema="{\"entries\":[{\"content\":{\"headerSize\":26,\"margin\":15,\"minimumSpacing\":25,\"sides\":[{\"content\":{\"connectorIds\":[]},\"type\":\"ConnectorPlacement.EquallySpacedRectSide\",\"uuid\":\"d6b19c1a-8540-4fb3-b3a7-b181a93e2dcd\"},{\"content\":{\"connectorIds\":[\"Out1\"],\"side\":\"RIGHT\"},\"type\":\"ConnectorPlacement.EquallySpacedRectSide\",\"uuid\":\"919fe610-1017-4d7e-ba89-b997ed30f941\"},{\"content\":{\"connectorIds\":[],\"side\":\"TOP\"},\"type\":\"ConnectorPlacement.EquallySpacedRectSide\",\"uuid\":\"6473f4db-e183-4279-8b70-07d1c7c027c3\"}]},\"type\":\"ConnectorPlacement.EquallySpacedConnector\",\"uuid\":\"f0cd8fda-dd3e-48df-a1f9-a7820f464db5\"}],\"packageUris\":[\"http://schema.mathworks.com/mf0/Connector/R2020b\"],\"version\":\"1.0\"}"
  X,Y Feedback : Subsystem
      settings: PortSchema="{\"entries\":[{\"content\":{\"headerSize\":26,\"margin\":15,\"minimumSpacing\":25,\"sides\":[{\"content\":{\"connectorIds\":[\"Out1\"]},\"type\":\"ConnectorPlacement.EquallySpacedRectSide\",\"uuid\":\"d6b19c1a-8540-4fb3-b3a7-b181a93e2dcd\"},{\"content\":{\"connectorIds\":[\"In1\"],\"side\":\"RIGHT\"},\"type\":\"ConnectorPlacement.EquallySpacedRectSide\",\"uuid\":\"919fe610-1017-4d7e-ba89-b997ed30f941\"},{\"content\":{\"connectorIds\":[],\"side\":\"TOP\"},\"type\":\"ConnectorPlacement.EquallySpacedRectSide\",\"uuid\":\"6473f4db-e183-4279-8b70-07d1c7c027c3\"}]},\"type\":\"ConnectorPlacement.EquallySpacedConnector\",\"uuid\":\"f0cd8fda-dd3e-48df-a1f9-a7820f464db5\"}],\"packageUris\":[\"http://schema.mathworks.com/mf0/Connector/R2020b\"],\"version\":\"1.0\"}"
  Bus Element Out2 : Outport  PortName=Pitch_Out
  Bus Element Out1 : Outport  Port=2  PortName=Roll_Out
  wires:
  Postion Reference/1(Reference) -> Adapter/2(Reference)
  X,Y Feedback/1(Feedback_Ref) -> Adapter/1(Feedback_Ref)
  Position Controller/1(Roll_Out) -> Bus Element Out1/1
  Position Controller/2(Pitch_Out) -> Bus Element Out2/1
  Bus Element In1/1 -> X,Y Feedback/1(FeedBack_Position)
  Adapter/1(X_Y_Info) -> Position Controller/1(X_Y_Info)

== system FlightControlArchitecture/Roll PID ==
  Bus Element In1 : Inport  PortName=R_Result
  Bus Element Out1 : Outport  PortName=Roll

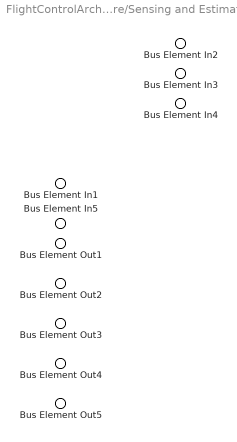
== system FlightControlArchitecture/Sensing and Estimation ==
  Bus Element In4 : Inport  PortName=Thrust_in
  Bus Element In3 : Inport  Port=2  PortName=Yaw_in
  Bus Element In2 : Inport  Port=3  PortName=Pitch_in
  Bus Element In1 : Inport  Port=4  PortName=Roll_in
  Bus Element In5 : Inport  Port=5  PortName=Position_in
  Bus Element Out1 : Outport  PortName=Thrust_est
  Bus Element Out2 : Outport  Port=2  PortName=Yaw_est
  Bus Element Out3 : Outport  Port=3  PortName=Pitch_est
  Bus Element Out4 : Outport  Port=4  PortName=Roll_est
  Bus Element Out5 : Outport  Port=5  PortName=Position_est

== system FlightControlArchitecture/Thrust PID ==
  Bus Element In1 : Inport  PortName=T_Result
  Bus Element Out1 : Outport  PortName=Thrust

== system FlightControlArchitecture/Yaw Angle ==
  Bus Element Out1 : Outport  PortName=Constant

== system FlightControlArchitecture/Yaw PID ==
  Bus Element In1 : Inport  PortName=Y_Result
  Bus Element Out1 : Outport  PortName=Yaw

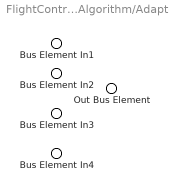
== system FlightControlArchitecture/Motor Mixing Algorithm/Adapter ==
  Bus Element In2 : Inport  PortName=P_out
  Bus Element In1 : Inport  Port=2  PortName=R_out
  Bus Element In3 : Inport  Port=3  PortName=Y_out
  Bus Element In4 : Inport  Port=4  PortName=T_out
  Out Bus Element : Outport  PortName=CMD_out

== system FlightControlArchitecture/Motor Mixing Algorithm/P ==
  Bus Element In1 : Inport  PortName=Pitch
  Bus Element Out1 : Outport  PortName=P_out

== system FlightControlArchitecture/Motor Mixing Algorithm/R ==
  Bus Element In1 : Inport  PortName=Roll
  Bus Element Out1 : Outport  PortName=R_out

== system FlightControlArchitecture/Motor Mixing Algorithm/T ==
  Bus Element In1 : Inport  PortName=Roll
  Bus Element Out1 : Outport  PortName=T_out

== system FlightControlArchitecture/Motor Mixing Algorithm/Y ==
  Bus Element In1 : Inport  PortName=Roll
  Bus Element Out1 : Outport  PortName=Y_out

== system FlightControlArchitecture/Outputs/Pitch_Feedback ==
  Bus Element Out1 : Outport  PortName=P_Feedback

== system FlightControlArchitecture/Outputs/Position_Feedback ==
  Bus Element Out1 : Outport  PortName=XY_Feedback

== system FlightControlArchitecture/Outputs/Roll_Feedback ==
  Bus Element Out1 : Outport  PortName=R_Feedback

== system FlightControlArchitecture/Outputs/Thrust_Feedback ==
  Bus Element Out1 : Outport  PortName=T_Feedback

== system FlightControlArchitecture/Outputs/Yaw_Feedback ==
  Bus Element Out1 : Outport  PortName=Y_Feedback

== system FlightControlArchitecture/Position Error Controller(Counteracts drifting of the drone)/Adapter ==
  Bus Element In1 : Inport  PortName=Feedback_Ref
  In Bus Element : Inport  Port=2  PortName=Reference
  Out Bus Element : Outport  PortName=X_Y_Info
  wires:
  In Bus Element/1 -> Out Bus Element/1

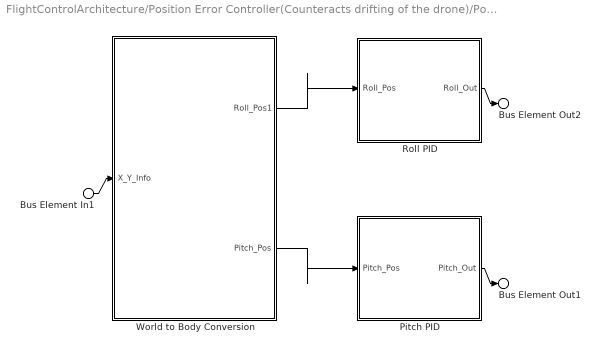
== system FlightControlArchitecture/Position Error Controller(Counteracts drifting of the drone)/Position Controller ==
  Bus Element In1 : Inport  PortName=X_Y_Info
  Pitch PID : Subsystem
      settings: PortSchema="{\"entries\":[{\"content\":{\"headerSize\":26,\"margin\":15,\"minimumSpacing\":25,\"sides\":[{\"content\":{\"connectorIds\":[\"In1\"]},\"type\":\"ConnectorPlacement.EquallySpacedRectSide\",\"uuid\":\"d6b19c1a-8540-4fb3-b3a7-b181a93e2dcd\"},{\"content\":{\"connectorIds\":[\"Out1\"],\"side\":\"RIGHT\"},\"type\":\"ConnectorPlacement.EquallySpacedRectSide\",\"uuid\":\"919fe610-1017-4d7e-ba89-b997ed30f941\"},{\"content\":{\"connectorIds\":[],\"side\":\"TOP\"},\"type\":\"ConnectorPlacement.EquallySpacedRectSide\",\"uuid\":\"6473f4db-e183-4279-8b70-07d1c7c027c3\"}]},\"type\":\"ConnectorPlacement.EquallySpacedConnector\",\"uuid\":\"f0cd8fda-dd3e-48df-a1f9-a7820f464db5\"}],\"packageUris\":[\"http://schema.mathworks.com/mf0/Connector/R2020b\"],\"version\":\"1.0\"}"
  Roll PID : Subsystem
      settings: PortSchema="{\"entries\":[{\"content\":{\"headerSize\":26,\"margin\":15,\"minimumSpacing\":25,\"sides\":[{\"content\":{\"connectorIds\":[\"In1\"]},\"type\":\"ConnectorPlacement.EquallySpacedRectSide\",\"uuid\":\"d6b19c1a-8540-4fb3-b3a7-b181a93e2dcd\"},{\"content\":{\"connectorIds\":[\"Out1\"],\"side\":\"RIGHT\"},\"type\":\"ConnectorPlacement.EquallySpacedRectSide\",\"uuid\":\"919fe610-1017-4d7e-ba89-b997ed30f941\"},{\"content\":{\"connectorIds\":[],\"side\":\"TOP\"},\"type\":\"ConnectorPlacement.EquallySpacedRectSide\",\"uuid\":\"6473f4db-e183-4279-8b70-07d1c7c027c3\"}]},\"type\":\"ConnectorPlacement.EquallySpacedConnector\",\"uuid\":\"f0cd8fda-dd3e-48df-a1f9-a7820f464db5\"}],\"packageUris\":[\"http://schema.mathworks.com/mf0/Connector/R2020b\"],\"version\":\"1.0\"}"
  World to Body Conversion : Subsystem
      settings: PortSchema="{\"entries\":[{\"content\":{\"headerSize\":26,\"margin\":15,\"minimumSpacing\":25,\"sides\":[{\"content\":{\"connectorIds\":[\"In1\"]},\"type\":\"ConnectorPlacement.EquallySpacedRectSide\",\"uuid\":\"d6b19c1a-8540-4fb3-b3a7-b181a93e2dcd\"},{\"content\":{\"connectorIds\":[\"Out1\",\"Out2\"],\"side\":\"RIGHT\"},\"type\":\"ConnectorPlacement.EquallySpacedRectSide\",\"uuid\":\"919fe610-1017-4d7e-ba89-b997ed30f941\"},{\"content\":{\"connectorIds\":[],\"side\":\"TOP\"},\"type\":\"ConnectorPlacement.EquallySpacedRectSide\",\"uuid\":\"6473f4db-e183-4279-8b70-07d1c7c027c3\"},{\"content\":{\"connectorIds\":[],\"side\":\"BOTTOM\"},\"type\":\"ConnectorPlacement.EquallySpacedRectSide\",\"uuid\":\"50f31339-066d-4b1a-9393-c0b51843fa85\"}]},\"type\":\"ConnectorPlacement.EquallySpacedConnector\",\"uuid\":\"f0cd8fda-dd3e-48df-a1f9-a7820f464db5\"}],\"packageUris\":[\"http://schema.mathworks.com/mf0/Connector/R2020b\"],\"version\":\"1.0\"}"
  Bus Element Out2 : Outport  PortName=Roll_Out
  Bus Element Out1 : Outport  Port=2  PortName=Pitch_Out
  wires:
  World to Body Conversion/2(Pitch_Pos) -> Pitch PID/1(Pitch_Pos)
  World to Body Conversion/1(Roll_Pos1) -> Roll PID/1(Roll_Pos)
  Pitch PID/1(Pitch_Out) -> Bus Element Out1/1
  Roll PID/1(Roll_Out) -> Bus Element Out2/1
  Bus Element In1/1 -> World to Body Conversion/1(X_Y_Info)

== system FlightControlArchitecture/Position Error Controller(Counteracts drifting of the drone)/Postion Reference ==
  Bus Element Out1 : Outport  PortName=Reference

== system FlightControlArchitecture/Position Error Controller(Counteracts drifting of the drone)/X,Y Feedback ==
  Bus Element In1 : Inport  PortName=FeedBack_Position
  Bus Element Out1 : Outport  PortName=Feedback_Ref

== system FlightControlArchitecture/Position Error Controller(Counteracts drifting of the drone)/Position Controller/Pitch PID ==
  Bus Element In1 : Inport  PortName=Pitch_Pos
  Bus Element Out1 : Outport  PortName=Pitch_Out

== system FlightControlArchitecture/Position Error Controller(Counteracts drifting of the drone)/Position Controller/Roll PID ==
  Bus Element In1 : Inport  PortName=Roll_Pos
  Bus Element Out1 : Outport  PortName=Roll_Out

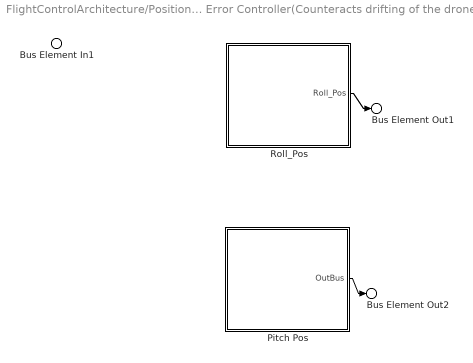
== system FlightControlArchitecture/Position Error Controller(Counteracts drifting of the drone)/Position Controller/World to Body Conversion ==
  Bus Element In1 : Inport  PortName=X_Y_Info
  Pitch Pos : Subsystem
      settings: PortSchema="{\"entries\":[{\"content\":{\"headerSize\":26,\"margin\":15,\"minimumSpacing\":25,\"sides\":[{\"content\":{\"connectorIds\":[]},\"type\":\"ConnectorPlacement.EquallySpacedRectSide\",\"uuid\":\"d6b19c1a-8540-4fb3-b3a7-b181a93e2dcd\"},{\"content\":{\"connectorIds\":[\"Out1\"],\"side\":\"RIGHT\"},\"type\":\"ConnectorPlacement.EquallySpacedRectSide\",\"uuid\":\"919fe610-1017-4d7e-ba89-b997ed30f941\"},{\"content\":{\"connectorIds\":[],\"side\":\"TOP\"},\"type\":\"ConnectorPlacement.EquallySpacedRectSide\",\"uuid\":\"6473f4db-e183-4279-8b70-07d1c7c027c3\"}]},\"type\":\"ConnectorPlacement.EquallySpacedConnector\",\"uuid\":\"f0cd8fda-dd3e-48df-a1f9-a7820f464db5\"}],\"packageUris\":[\"http://schema.mathworks.com/mf0/Connector/R2020b\"],\"version\":\"1.0\"}"
  Roll_Pos : Subsystem
      settings: PortSchema="{\"entries\":[{\"content\":{\"headerSize\":26,\"margin\":15,\"minimumSpacing\":25,\"sides\":[{\"content\":{\"connectorIds\":[]},\"type\":\"ConnectorPlacement.EquallySpacedRectSide\",\"uuid\":\"d6b19c1a-8540-4fb3-b3a7-b181a93e2dcd\"},{\"content\":{\"connectorIds\":[\"Out1\"],\"side\":\"RIGHT\"},\"type\":\"ConnectorPlacement.EquallySpacedRectSide\",\"uuid\":\"919fe610-1017-4d7e-ba89-b997ed30f941\"},{\"content\":{\"connectorIds\":[],\"side\":\"TOP\"},\"type\":\"ConnectorPlacement.EquallySpacedRectSide\",\"uuid\":\"6473f4db-e183-4279-8b70-07d1c7c027c3\"}]},\"type\":\"ConnectorPlacement.EquallySpacedConnector\",\"uuid\":\"f0cd8fda-dd3e-48df-a1f9-a7820f464db5\"}],\"packageUris\":[\"http://schema.mathworks.com/mf0/Connector/R2020b\"],\"version\":\"1.0\"}"
  Bus Element Out1 : Outport  PortName=Roll_Pos1
  Bus Element Out2 : Outport  Port=2  PortName=Pitch_Pos
  wires:
  Pitch Pos/1(OutBus) -> Bus Element Out2/1
  Roll_Pos/1(Roll_Pos) -> Bus Element Out1/1

== system FlightControlArchitecture/Position Error Controller(Counteracts drifting of the drone)/Position Controller/World to Body Conversion/Pitch Pos ==
  Bus Element Out1 : Outport  PortName=OutBus

== system FlightControlArchitecture/Position Error Controller(Counteracts drifting of the drone)/Position Controller/World to Body Conversion/Roll_Pos ==
  Bus Element Out1 : Outport  PortName=Roll_Pos
